simulink model "BlocosArredondamento"  (Simulink 5.0)
settings: Solver=ode45  StartTime=0.0  StopTime=10.0  RelTol=1e-3
values from neighbouring files (symbols this model uses):
  Ap = [      0    0.4758   -0.0018   -0.0000 ... (first row only)    [Arredondamento.m]
  Bp = [ 0.0404 ; -0.0404 ; -0.7709 ; 0]    [Arredondamento.m]
  Cp = [1 0 0 0]    [Arredondamento.m]
  Hp = [0 0 0 1]    [Arredondamento.m]    (also in RollYaw.m = u*sin(theta)          - v*cos(theta)*sin(fi)                )
  kd = K(3)    [Arredondamento.m]
  ki = K(2)    [Arredondamento.m]
  kp = K(1)    [Arredondamento.m]
  kr = K(5)    [Arredondamento.m]
  kt = K(4)    [Arredondamento.m]
  x0 = [-2.5*pi/180 0 0 16]    [Arredondamento.m]    (also in ClimbIas.m = X(5); LongitudinalAP.m = X(6); LongitudinalSAS.m = X(6); RollYaw.m = X(10))
libraries: simulink_extras x1
settings Model: LastModifiedBy=Tom

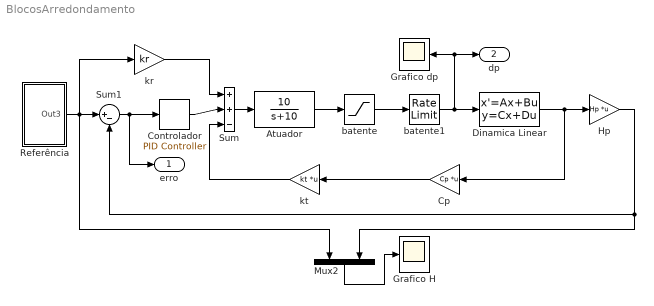
== system BlocosArredondamento ==
  Atuador : TransferFcn  Numerator=[10]  Denominator=[1 10]
  "Controlador " : simulink_extras/Additional Linear/PID Controller  P=kp  I=ki  D=kd
  Cp : Gain  Orientation=left  Gain=Cp  Multiplication=Matrix(K*u)  SaturateOnIntegerOverflow=on
  Dinamica Linear : StateSpace  A=Ap  B=Bp  C=eye(size(Ap))  D=zeros(size(Bp))  X0=x0
  Grafico H : Scope
      settings: TimeRange=20  YMin=0  YMax=16
  Grafico dp : Scope
  Hp : Gain  Gain=Hp  Multiplication=Matrix(K*u)  SaturateOnIntegerOverflow=on
  Mux2 : Mux  Orientation=down  Inputs=2
  Referência : Subsystem
  Sum : Sum  Inputs=|++-  SaturateOnIntegerOverflow=on
  Sum1 : Sum  Inputs=|+-  SaturateOnIntegerOverflow=on  InputSameDT=on
  batente : Saturate  UpperLimit=30  LowerLimit=-30
  batente1 : RateLimiter  RisingSlewLimit=60  FallingSlewLimit=-60
  kr : Gain  Gain=kr  SaturateOnIntegerOverflow=on
  kt : Gain  Orientation=left  Gain=kt  Multiplication=Matrix(K*u)  SaturateOnIntegerOverflow=on
  erro : Outport
  dp : Outport  Port=2
  wires:
  batente1/1 -> Dinamica Linear/1, dp/1, Grafico dp/1
  batente/1 -> batente1/1
  Atuador/1 -> batente/1
  Sum/1 -> Atuador/1
  "Controlador "/1 -> Sum/2
  Sum1/1 -> "Controlador "/1, erro/1
  Referência/1(Out3) -> Sum1/1, kr/1, Mux2/1
  Dinamica Linear/1 -> Hp/1, Cp/1
  Cp/1 -> kt/1
  kt/1 -> Sum/3
  kr/1 -> Sum/1
  Hp/1 -> Mux2/2, Sum1/2
  Mux2/1 -> Grafico H/1

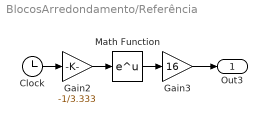
== system BlocosArredondamento/Referência ==
  Clock : Clock
      settings: Decimation=10
  Gain2 : Gain  Gain=-1/3.333  SaturateOnIntegerOverflow=on
  Gain3 : Gain  Gain=16  SaturateOnIntegerOverflow=on
  Math Function : Math
  Out3 : Outport
  wires:
  Gain3/1 -> Out3/1
  Gain2/1 -> Math Function/1
  Math Function/1 -> Gain3/1
  Clock/1 -> Gain2/1
